simulink model "OneWheelVehicleModel"  (Simulink 9.1)
settings: Solver=VariableStepAuto  StartTime=0.0  StopTime=20  FixedStep=1e-4  MaxStep=1e-2  RelTol=1e-3
values from neighbouring files (symbols this model uses):
  Kv = 0.5    [SimWheelVehicle.m]
  Kw = 100    [SimWheelVehicle.m]
  m = 200    [SimWheelVehicle.m]
  mwe = 1    [SimWheelVehicle.m]
  T = 0.01    [SimWheelVehicle.m]
  T0 = 0.004    [SimWheelVehicle.m]
settings Model: Creator=mb2287  LastModifiedBy=mb2287
settings DataIOCC: SaveFormat=Dataset
settings OptimizationCC: LifeSpan=auto
settings DebuggingCC: UnderspecifiedInitializationDetection=Simplified  MergeDetectMultiDrivingBlocksExec=error  LibraryContextMissingDiagnostic=warning  SFUnexpectedBacktrackingDiag=error  SFNoUnconditionalDefaultTransitionDiag=error  SFExecutionAtInitializationDiag=warning
settings HardwareCC: ProdBitPerPointer=64  ProdBitPerSizeT=64  ProdBitPerPtrDiffT=64  ProdLargestAtomicFloat=Float  ProdIntDivRoundTo=Zero  ProdEndianess=LittleEndian  ProdWordSize=64  ProdHWDeviceType=Intel->x86-64 (Windows64)
settings ModelReferenceCC: PropagateSignalLabelsOutOfModel=on
settings SFSimCC: SimUseLocalCustomCode=on
settings RTWCC: RTWUseLocalCustomCode=on
settings CodeAppCC: StateflowObjectComments=off
settings GRTTargetCC: TargetLangStandard=C99 (ISO)  CombineOutputUpdateFcns=on  GRTInterface=off
settings ConfigComp: CovMetricSettings=dwe  CovHtmlReporting=off  CovSaveCumulativeToWorkspaceVar=off  CovSaveSingleToWorkspaceVar=off  CovExternalEMLEnable=on

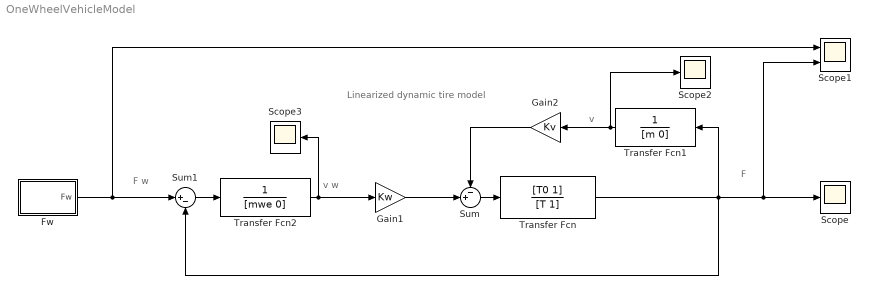
== system OneWheelVehicleModel ==
  note: v w
  note: v
  note: F
  note: F w
  note: Linearized dynamic tire model
  Fw : Subsystem
  Gain1 : Gain  Gain=Kw
  Gain2 : Gain  Gain=Kv
  Scope : Scope
  Scope1 : Scope  NumInputPorts=2
  Scope2 : Scope
  Scope3 : Scope
  Sum : Sum  Inputs=-+|
  Sum1 : Sum  Inputs=|+-
  Transfer Fcn : TransferFcn  Numerator=[T0 1]  Denominator=[T 1]
  Transfer Fcn1 : TransferFcn  Denominator=[m 0]
  Transfer Fcn2 : TransferFcn  Denominator=[mwe 0]
  wires:
  Fw/1(Fw) -> Scope1/1, Sum1/1
  Transfer Fcn1/1 -> Scope2/1, Gain2/1
  Transfer Fcn2/1 -> Scope3/1, Gain1/1
  Sum1/1 -> Transfer Fcn2/1
  Sum/1 -> Transfer Fcn/1
  Transfer Fcn/1 -> Sum1/2, Scope1/2, Scope/1, Transfer Fcn1/1
  Gain1/1 -> Sum/2
  Gain2/1 -> Sum/1

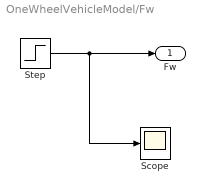
== system OneWheelVehicleModel/Fw ==
  Scope : Scope
  Step : Step  Time=10  Before=1000  After=2000  SampleTime=0
  Fw : Outport
  wires:
  Step/1 -> Scope/1, Fw/1
